simulink model "sensor_fault_profiles_for_current"  (Simulink 7.9)
settings: Solver=ode45  StartTime=0.0  StopTime=10.0  RelTol=1e-3
values from neighbouring files (symbols this model uses):
  current_fault_time = 7    [check_time_with_lqg_and_nn.m]    (also in current_inc_abr.m = 1; fault_tests_abrupt_add_igva_iFD.m = 2; fault_tests_abrupt_add_igva_lqgFD.m = 2; fault_tests_abrupt_bias_igva_iFD.m = 2)
  fault_type_i = 1    [check_time_with_lqg_and_nn.m]    (also in current_inc_abr.m = 2; fault_tests_abrupt_add_igva_iFD.m = 2; fault_tests_abrupt_add_igva_lqgFD.m = 2; fault_tests_abrupt_bias_igva_iFD.m = 5)
  i_slope = -0.8    [check_time_with_lqg_and_nn.m]    (also in current_inc_abr.m; fault_tests_abrupt_add_igva_iFD.m = 20; fault_tests_abrupt_add_igva_lqgFD.m = 20; fault_tests_abrupt_bias_igva_iFD.m)
  Tsamp = 0.001    [LSDP_controllers_nntraining_data_igva.m]    (also in initialize_LSDP_controllers_igva.m)
libraries: simulink x5
settings Model: Creator=kostas  LastModifiedBy=kostas

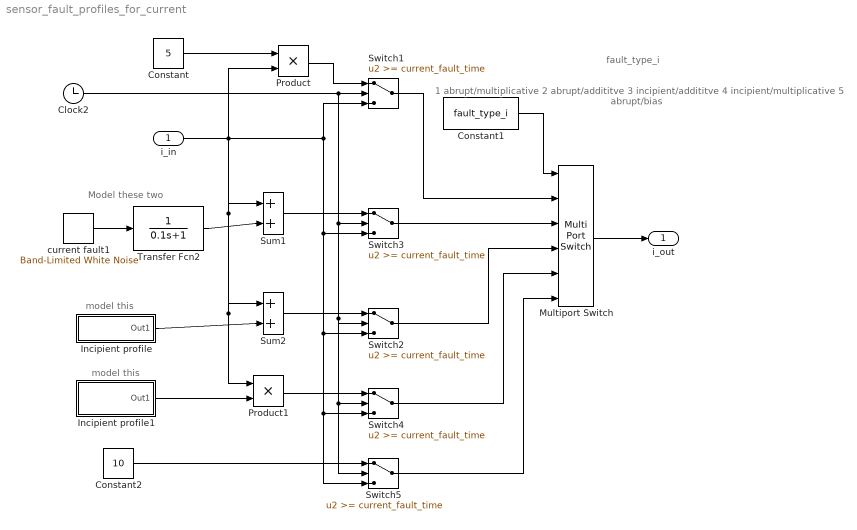
== system sensor_fault_profiles_for_current ==
  note: 1 abrupt/multiplicative
      | 2 abrupt/addititve
      | 3 incipient/addititve
      | 4 incipient/multiplicative
      | 5 abrupt/bias
  note: fault_type_i
  note: model this
  note: model this
  note: Model these two
  i_in : Inport
  Clock2 : Clock
  Constant : Constant  Value=5
  Constant1 : Constant  Value=fault_type_i
  Constant2 : Constant  Value=10
  Incipient profile : Subsystem
  Incipient profile1 : Subsystem
  Multiport Switch : MultiPortSwitch  Inputs=5  zeroidx=off
  Product : Product  RndMeth=Zero
  Product1 : Product  RndMeth=Zero
  Sum1 : Sum  Inputs=|++
  Sum2 : Sum  Inputs=|++
  Switch{1..5} (5 alike) : Switch  Threshold=current_fault_time
  Transfer Fcn2 : TransferFcn  Denominator=[0.1 1]
  current fault1 : simulink/Sources/Band-Limited White Noise  Cov=5  Ts=Tsamp  seed=[24353]
  i_out : Outport
  wires:
  i_in/1 -> Switch1/3, Switch3/3, Switch2/3, Switch4/3, Switch5/3, Sum1/1, Sum2/1, Product1/1, Product/2
  Clock2/1 -> Switch1/2, Switch3/2, Switch2/2, Switch4/2, Switch5/2
  Constant/1 -> Product/1
  Multiport Switch/1 -> i_out/1
  Switch1/1 -> Multiport Switch/2
  Constant1/1 -> Multiport Switch/1
  Sum1/1 -> Switch3/1
  Switch3/1 -> Multiport Switch/3
  Product/1 -> Switch1/1
  current fault1/1 -> Transfer Fcn2/1
  Transfer Fcn2/1 -> Sum1/2
  Sum2/1 -> Switch2/1
  Switch2/1 -> Multiport Switch/4
  Switch4/1 -> Multiport Switch/5
  Constant2/1 -> Switch5/1
  Product1/1 -> Switch4/1
  Incipient profile1/1(Out1) -> Product1/2
  Switch5/1 -> Multiport Switch/6
  Incipient profile/1(Out1) -> Sum2/2

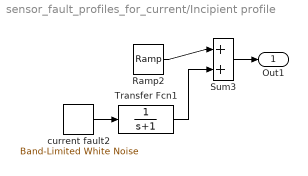
== system sensor_fault_profiles_for_current/Incipient profile ==
  Ramp2 : simulink/Sources/Ramp  slope=i_slope  start=current_fault_time  X0=0
  Sum3 : Sum  Inputs=|++
  Transfer Fcn1 : TransferFcn  Numerator=1  Denominator=[1 1]
  current fault2 : simulink/Sources/Band-Limited White Noise  Cov=1  Ts=Tsamp  seed=[21351]
  Out1 : Outport
  wires:
  current fault2/1 -> Transfer Fcn1/1
  Ramp2/1 -> Sum3/1
  Sum3/1 -> Out1/1
  Transfer Fcn1/1 -> Sum3/2

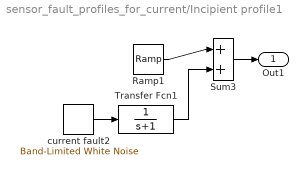
== system sensor_fault_profiles_for_current/Incipient profile1 ==
  Ramp1 : simulink/Sources/Ramp  slope=i_slope  start=current_fault_time  X0=1
  Sum3 : Sum  Inputs=|++
  Transfer Fcn1 : TransferFcn  Denominator=[1 1]
  current fault2 : simulink/Sources/Band-Limited White Noise  Cov=1  Ts=Tsamp  seed=[23341]
  Out1 : Outport
  wires:
  Sum3/1 -> Out1/1
  Transfer Fcn1/1 -> Sum3/2
  Ramp1/1 -> Sum3/1
  current fault2/1 -> Transfer Fcn1/1
